simulink subsystem "FanModule_2025a"  (R2025a)
settings: Solver=VariableStepAuto  StartTime=0.0  StopTime=10.0  RelTol=1e-3
model mask{min_fan_speed=0.05, tau=0.1, max_thrust=3.53, radius=0.5, max_speed=62500}
  mask prompts: min_fan_speed "min Fan Speed (%)"; tau "Time Constant (s)"; max_thrust "Max Thrust (N)"; radius "Radius (m)"; max_speed "Max Speed (RPM)"
settings Model: Creator=wangzerun  LastModifiedBy=wangzerun

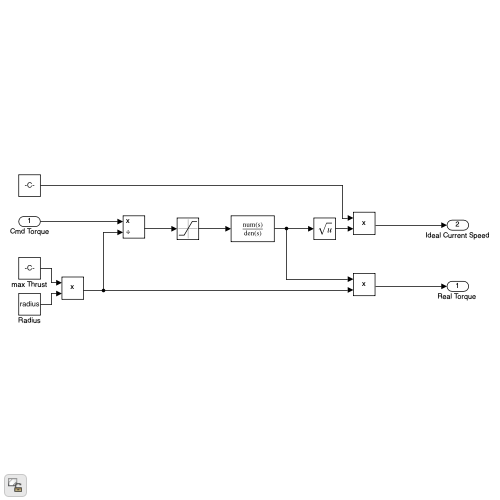
[thumbnail: Simulink's stored preview of the top-level diagram]
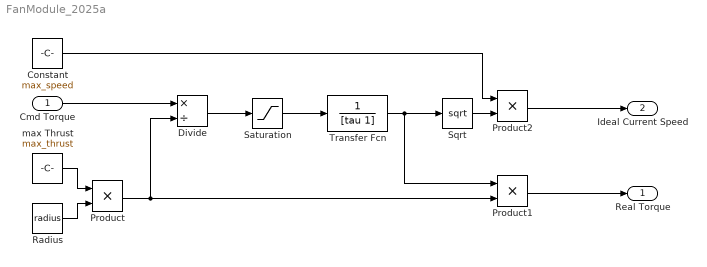
== system FanModule_2025a ==
  Cmd Torque : Inport
  Constant : Constant  Value=max_speed
  Divide : Product  Inputs=*/
  Product : Product
  Product1 : Product
  Product2 : Product
  Radius : Constant  Value=radius
  Saturation : Saturate  UpperLimit=1  LowerLimit=min_fan_speed
  Sqrt : Sqrt
  Transfer Fcn : TransferFcn  Denominator=[tau 1]
  max Thrust : Constant  Value=max_thrust
  "Real Torque " : Outport
  Ideal Current Speed : Outport  Port=2
  wires:
  Transfer Fcn/1 -> Sqrt/1, Product1/1
  Saturation/1 -> Transfer Fcn/1
  Cmd Torque/1 -> Divide/1
  Divide/1 -> Saturation/1
  max Thrust/1 -> Product/1
  Radius/1 -> Product/2
  Product/1 -> Product1/2, Divide/2
  Product1/1 -> "Real Torque "/1
  Sqrt/1 -> Product2/2
  Constant/1 -> Product2/1
  Product2/1 -> Ideal Current Speed/1
